simulink subsystem "muscle_dynamics_subsystem"  (R2020a)
settings: Solver=VariableStepAuto  StartTime=0.0  StopTime=10.0  RelTol=1e-3
undefined symbols (not defined in the file): T_stim
settings Model: Creator=jmei13  LastModifiedBy=jmei13

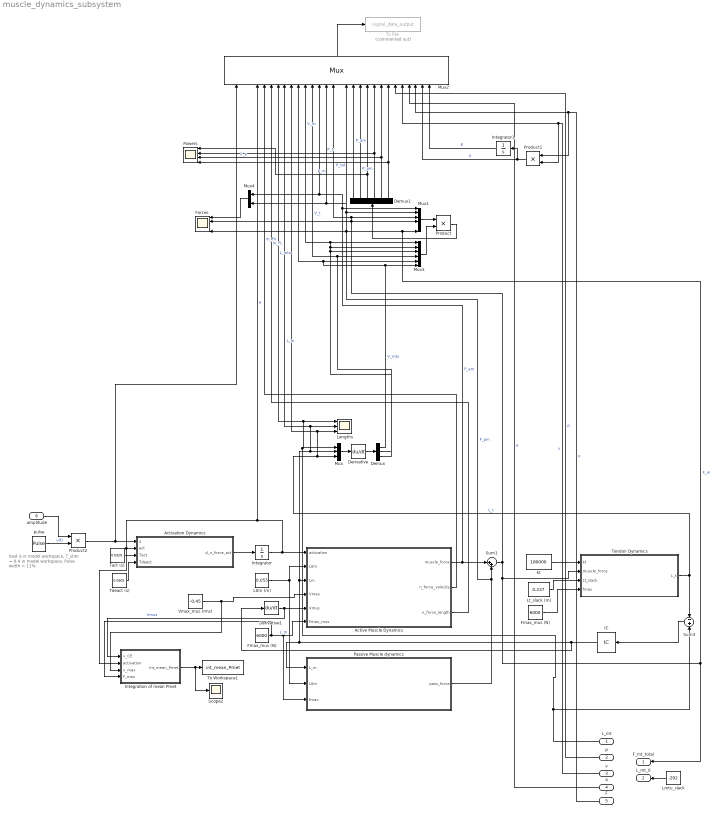
== system muscle_dynamics_subsystem ==
  note: load is in model workspace,
      | T_stim = 0.4 in model workspace,
      | Pulse width = 11%
  L_mt : Inport
  p : Inport  Port=2
  v : Inport  Port=3
  a : Inport  Port=4
  F : Inport  Port=5
  amplitude : Inport  Port=6
  Activation Dynamics : MATLAB Function  TreatAsAtomicUnit=on
  Active Muscle Dynamics : MATLAB Function
  Demux : Demux  Outputs=3
  Demux1 : Demux  Outputs=6
  Derivative : Derivative
  Derivative1 : Derivative
  Fmax_mus (N) : Constant  Value=6000
  "Fmax_mus (N) " : Constant  Value=6000
  Forces : Scope  NumInputPorts=4
  IC : InitialCondition  Value=0.055
  Integration of mean Pmet : Subsystem
  Integrator : Integrator
  Integrator1 : Integrator
  L0m (m) : Constant  Value=0.055
  Lengths : Scope  NumInputPorts=3
  Lmtu_slack : Constant  Value=.292
  Lt_slack (m) : Constant  Value=0.237
  Mux : Mux  Inputs=3
  Mux1 : Mux  Inputs=6
  Mux2 : Mux  Inputs=30
      settings: DisplayOption=signals
  Mux3 : Mux  Inputs=6
  Mux4 : Mux  Inputs=2
  Passive Muscle dynamics : MATLAB Function
  Powers : Scope  NumInputPorts=4
  Product : Product
  Product1 : Product
  Product2 : Product
  Scope2 : Scope
  Sum1 : Sum  Inputs=|++
  Sum3 : Sum  Inputs=-|+
  Tact (s) : Constant  Value=0.0329  VectorParams1D=off
  Tdeact (s) : Constant  Value=0.0905
  Tendon Dynamics : MATLAB Function
  To File : ToFile  Commented=on  Filename=signal_data_output  MatrixName=data  SaveFormat=Timeseries
  To Workspace1 : ToWorkspace  VariableName=int_mean_Pmet  SaveFormat=Timeseries  SampleTime=-1
  Vmax_mus (m\s) : Constant  Value=-0.45
  kt : Constant  Value=180000
  pulse : DiscretePulseGenerator  PulseType=Time based  Period=T_stim  PulseWidth=11
  F_mt_total : Outport
  L_mt_0 : Outport  Port=2
  wires:
  Mux4/1 -> Forces/1
  Integrator1/1 -> Mux2/29  "E"
  L0m (m)/1 -> Active Muscle Dynamics/2(L0m), Passive Muscle dynamics/2(L0m)  "L_m"
  Mux2/1 -> To File/1
  v/1 -> Product1/2, Mux2/25  "v"
  Tact (s)/1 -> Activation Dynamics/3(Tact)
  Mux1/1 -> Product/1
  p/1 -> Mux2/24  "p"
  Demux1/6 -> Mux2/23, Powers/4  "P_tot"
  Lmtu_slack/1 -> L_mt_0/1
  Demux1/4 -> Mux2/21, Powers/2  "P_t"
  Demux1/3 -> Mux2/20, Powers/1  "P_m"
  Demux1/5 -> Mux2/22, Powers/3  "P_e"
  Active Muscle Dynamics/2(n_force_velocity) -> Mux2/5  "m_FV"
  Mux/1 -> Derivative/1
  Passive Muscle dynamics/1(pass_force) -> Mux1/2, Mux4/2, Mux2/14, Sum1/2  "F_pm"
  Derivative/1 -> Demux/1
  kt/1 -> Tendon Dynamics/1(kt)
  Demux1/1 -> Mux2/18  "P_am"
  Vmax_mus (m\s)/1 -> Integration of mean Pmet/3(v_max), Active Muscle Dynamics/4(Vmax)
  Demux1/2 -> Mux2/19  "P_pm"
  Active Muscle Dynamics/3(n_force_length) -> Mux2/6  "m_FL"
  Sum1/1 -> Mux1/4, Mux1/3, Mux2/15, Forces/2, F_mt_total/1, Mux1/6, Forces/4, Mux2/17, Tendon Dynamics/2(muscle_force)  "F_m"
  pulse/1 -> Product2/2  "u(t)"
  a/1 -> Mux2/26  "a"
  Lt_slack (m)/1 -> Tendon Dynamics/3(Lt_slack)
  Demux/1 -> Mux3/5, Mux2/10, Mux3/6  "V_mtu"
  Demux/3 -> Mux3/4, Mux2/12  "V_t"
  Tdeact (s)/1 -> Activation Dynamics/4(Tdeact)
  Activation Dynamics/1(d_n_force_act) -> Integrator/1
  Product1/1 -> Mux2/28, Integrator1/1  "P"
  Product/1 -> Demux1/1
  "Fmax_mus (N) "/1 -> Tendon Dynamics/4(fmax)
  Active Muscle Dynamics/1(muscle_force) -> Sum1/1, Mux1/1, Mux4/1, Mux2/13  "F_am"
  L_mt/1 -> Sum3/2, Lengths/1, Mux2/7, Mux/1  "L_mtu"
  Fmax_mus (N)/1 -> Integration of mean Pmet/4(F_max), Passive Muscle dynamics/3(fmax), Active Muscle Dynamics/6(Fmax_mus)
  Mux3/1 -> Product/2
  Tendon Dynamics/1(L_t) -> Lengths/3, Mux2/9, Mux/3, Sum3/1  "L_t"
  Derivative1/1 -> Integration of mean Pmet/1(v_CE), Active Muscle Dynamics/5(Vmus)  "Vmus"
  Demux/2 -> Mux3/3, Mux3/2, Mux3/1, Mux2/11  "V_m"
  F/1 -> Product1/1, Mux2/27  "F"
  Integrator/1 -> Active Muscle Dynamics/1(activation), Integration of mean Pmet/2(activation), Activation Dynamics/2(act), Mux2/4  "a"
  Integration of mean Pmet/1(Int_mean_Pmet) -> To Workspace1/1, Scope2/1
  Sum3/1 -> IC/1
  IC/1 -> Derivative1/1, Passive Muscle dynamics/1(L_m), Mux/2, Lengths/2, Mux2/8, Active Muscle Dynamics/3(Lm)  "L_m"
  amplitude/1 -> Product2/1
  Product2/1 -> Mux2/1, Activation Dynamics/1(u)

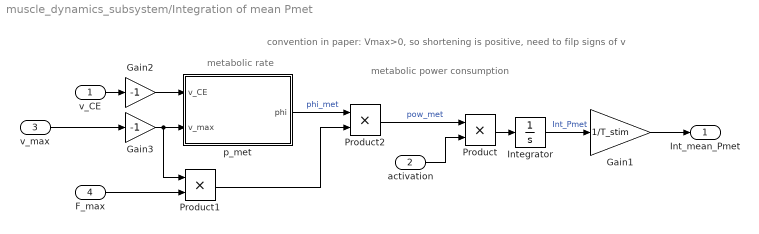
== system muscle_dynamics_subsystem/Integration of mean Pmet ==
  note: convention in paper: Vmax>0, so shortening is positive, need to filp signs of v
  note: metabolic power consumption
  note: metabolic rate
  v_CE : Inport
  activation : Inport  Port=2
  v_max : Inport  Port=3
  F_max : Inport  Port=4
  Gain1 : Gain  Gain=1/T_stim
  Gain2 : Gain  Gain=-1
  Gain3 : Gain  Gain=-1
  Integrator : Integrator
  Product : Product
  Product1 : Product
  Product2 : Product
  p_met : MATLAB Function  TreatAsAtomicUnit=on
  Int_mean_Pmet : Outport
  wires:
  v_CE/1 -> Gain2/1
  activation/1 -> Product/2
  Product/1 -> Integrator/1
  Integrator/1 -> Gain1/1  "Int_Pmet"
  Product2/1 -> Product/1  "pow_met"
  p_met/1(phi) -> Product2/1  "phi_met"
  Gain3/1 -> Product1/1, p_met/2(v_max)
  Gain1/1 -> Int_mean_Pmet/1
  Gain2/1 -> p_met/1(v_CE)
  v_max/1 -> Gain3/1
  F_max/1 -> Product1/2
  Product1/1 -> Product2/2

== matlab function muscle_dynamics_subsystem/Active Muscle Dynamics ==
  data: activation input; L0m input; Lm input; Vmax input; Vmus input; Fmax_mus input; muscle_force output; n_force_velocity output; n_force_length output
function [muscle_force, n_force_velocity, n_force_length]  =...
    muscle_dynamics(activation,L0m,Lm,Vmax,Vmus,Fmax_mus)
%#codegen

    %Hill Type Muscle F-V relationship.  Returns a normalized force-velocity value
    if (Vmus<Vmax)
        n_force_velocity=0;
    else
        if (Vmus >= Vmax && Vmus < 0)
            n_force_velocity = ((1-(Vmus/Vmax))/(1+(Vmus/0.17/Vmax)));
        else
            n_force_velocity =(1.8-0.8*((1+(Vmus/Vmax))/(1-7.56*Vmus/0.17/Vmax)));
        end
    end
    
    %Active muscle F-L relationships.  Returns a normalized F-L value

    a = 3.1108;
    b = .8698;
    s = .3914;

    if Lm < 0
        Lm = 0;
    end

    n_force_length = exp(-(abs(((Lm/L0m)^b-1)/s))^a);

    %Total active force of muscle based on normalized F-V and F-L relationships
    muscle_force = Fmax_mus* activation * n_force_velocity * n_force_length;
end

== matlab function muscle_dynamics_subsystem/Tendon Dynamics ==
  data: kt input; L_t output; muscle_force input; Lt_slack input; fmax input
function L_t = L_tendon(kt,muscle_force,Lt_slack,fmax)
%#codegen

%Total tendon length
%kt_comp = @(fm) 1./(kt*(1+(0.9./((-exp((20*fm)./fmax))))));
dL_t = ((muscle_force + (fmax*log((-9*exp(-(20*muscle_force)/fmax)) + 10))/20)/kt);
L_t = dL_t + Lt_slack ;

end

== matlab function muscle_dynamics_subsystem/Activation Dynamics ==
  data: u input; d_n_force_act output; act input; Tact input; Tdeact input
function d_n_force_act = d_n_force_act(u,act,Tact,Tdeact)
%#codegen    
%Rate of change of activation
    B=Tact/Tdeact;
    d_n_force_act= u/Tact - (1/Tact*(B+(1-B)*u))*act;
end

== matlab function muscle_dynamics_subsystem/Passive Muscle dynamics ==
  data: pass_force output; L_m input; L0m input; fmax input
function pass_force = pmuscle_dynamics(L_m, L0m,fmax)
%#codegen
%passive CE F_L taken from Rubenson et. al.

%Passive muscle force
A = 2.38*10^(-2);
b = 5.31;

if L_m > 0    
    pass_force= fmax*A*exp(b*((L_m/L0m)-1));
else
    pass_force=0;
end


end

== matlab function muscle_dynamics_subsystem/Integration of mean Pmet/p_met ==
  data: v_CE input; phi output; v_max input
function phi = p_met(v_CE, v_max)

if v_CE<0
    phi = 0.01 - 0.11*(v_CE/v_max) + 0.06*exp(23*v_CE/v_max);
else
    phi = 0.23 - 0.16*exp(-8*v_CE/v_max);
end
